simulink model "PMSM_9_yuanlei_SMO_atan_current_step_2019b"  (R2019b)
settings: Solver=ode3  StartTime=0.0  StopTime=0.35  FixedStep=2e-7  RelTol=1e-4  EnableMultiTasking=on
InitFcn:
  | R = 2.8750;
  | L = 8.5e-3;
libraries: powerlib x6, simulink x1
settings Model: Creator=Lei  LastModifiedBy=Administrator
settings DataIOCC: LimitDataPoints=on  SaveFormat=Array  ReturnWorkspaceOutputs=off
settings OptimizationCC: ExpressionDepthLimit=2147483647  InitFltsAndDblsToZero=on  LifeSpan=inf
settings DebuggingCC: SaveWithParameterizedLinksMsg=none  UnderspecifiedInitializationDetection=Classic  MergeDetectMultiDrivingBlocksExec=none  SignalResolutionControl=TryResolveAllWithWarning  SolverPrmCheckMsg=warning  MultiTaskDSMMsg=warning  MultiTaskCondExecSysMsg=none  FcnCallInpInsideContextMsg=warning  UnconnectedLineMsg=none  StateNameClashWarn=warning  SFUnexpectedBacktrackingDiag=warning  SFNoUnconditionalDefaultTransitionDiag=warning  SFExecutionAtInitializationDiag=none  ArithmeticOperatorsInVariantConditions=warning
settings HardwareCC: ProdBitPerPointer=32  ProdBitPerSizeT=32  ProdBitPerPtrDiffT=32  ProdLargestAtomicFloat=None  ProdIntDivRoundTo=Undefined  ProdEndianess=Unspecified  ProdWordSize=32  ProdHWDeviceType=32-bit Generic
settings ModelReferenceCC: PropagateSignalLabelsOutOfModel=off
settings SFSimCC: SimUseLocalCustomCode=off  CustomCodeUndefinedFunction=UseInterfaceOnly
settings RTWCC: RTWUseLocalCustomCode=off
settings CodeAppCC: StateflowObjectComments=on
settings GRTTargetCC: TargetFcnLib=ansi_tfl_tmw.mat  TargetLangStandard=C89/C90 (ANSI)  GeneratePreprocessorConditionals=Disable all  CombineOutputUpdateFcns=off  GRTInterface=on
settings ConfigComp: CovMetricSettings=dw  CovHtmlReporting=on  CovSaveCumulativeToWorkspaceVar=on  CovSaveSingleToWorkspaceVar=on  CovExternalEMLEnable=off  CovSFcnEnable=off
settings SimscapeCC: SimscapeNormalizeSystem=off

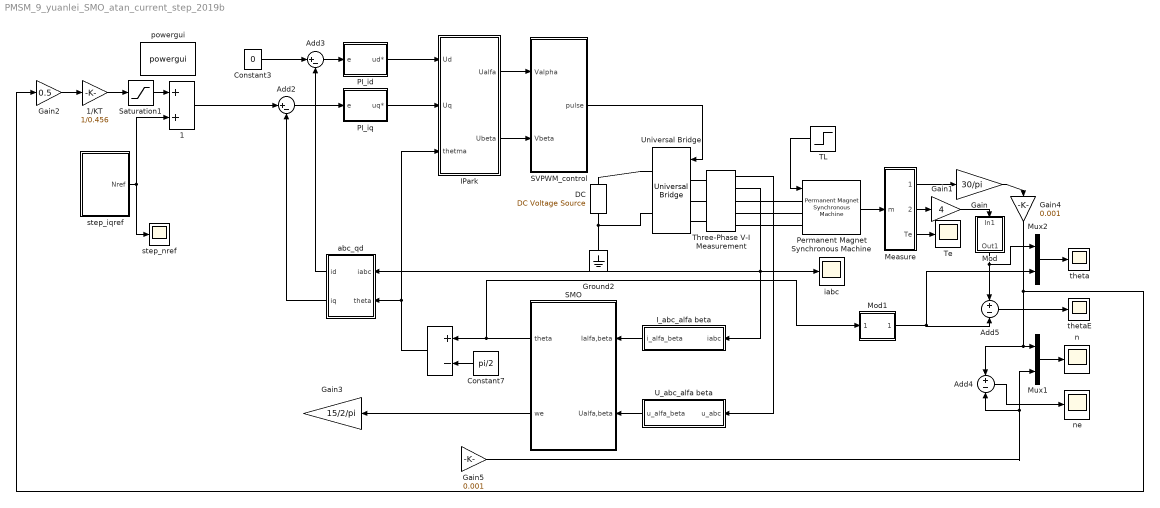
== system PMSM_9_yuanlei_SMO_atan_current_step_2019b ==
  "  " : Sum  Inputs=+-
  "  1" : Sum
  1/KT : Gain  Gain=1/0.456
  Add2 : Sum  Inputs=|+-
  Add3 : Sum  Inputs=|+-
  Add4 : Sum  Inputs=+|-
  Add5 : Sum  Inputs=+|-
  Constant3 : Constant  Value=0
  Constant7 : Constant  Value=pi/2
  "DC " : powerlib/Electrical Sources/DC Voltage Source  Amplitude=311  Measurements=None
      settings: SourceProductName=Simscape Electrical
  Gain : Gain  Gain=30/pi
  Gain1 : Gain  Gain=4
  Gain2 : Gain  Gain=0.5
  Gain3 : Gain  Gain=15/2/pi
  Gain4 : Gain  Gain=0.001
  Gain5 : Gain  Gain=0.001
  Ground2 : powerlib/Elements/Ground  LConnTagsString=a
      settings: SourceProductName=Simscape Electrical
  IPark : Subsystem
  I_abc_alfa beta : Subsystem
  Measure : Subsystem
  Mod : Subsystem
  Mod1 : Subsystem
  Mux1 : Mux  Inputs=2
  Mux2 : Mux  Inputs=2
  PI_id : Subsystem
      mask Display: disp('PI')
  PI_iq : Subsystem
      mask Display: disp('PI')
  Permanent Magnet Synchronous Machine : powerlib/Machines/Permanent Magnet Synchronous Machine  NbPhases=3  FluxDistribution=Sinusoidal  RotorType=Salient-pole  MechanicalLoad=Torque Tm  PresetModel=No  ShowDetailedParameters=on  MeasurementBus=off  Resistance=2.8750  Inductance=8.5e-3  dqInductances=[8.5e-3, 8.5e-3]  La=0.000835  MachineConstant=Flux linkage established by magnets (V.s)  Flux=0.175  VoltageCst=126.966  TorqueCst=1.05  Flat=120  Mechanical="[ 1e-3, 0,  4 ]"  PolePairs=4  InitialConditions=[0,0, 0,0]  InitialConditions5ph=[0 0 0 0 0 0]  RefAngle=90 degrees behind phase A axis (modified Park)  IterativeDiscreteModel=Trapezoidal non iterative  TsBlock=-1  TsPowergui=0
  SMO : Subsystem
  SVPWM_control : Subsystem
  Saturation1 : Saturate  UpperLimit=1  LowerLimit=-1
  TL : Step  Time=0  After=3  SampleTime=0
  Te : Scope
  Three-Phase V-I Measurement : powerlib/Measurements/Three-Phase V-I Measurement  VoltageMeasurement=phase-to-ground  SetLabelV=off  LabelV=Vabc  Vpu=off  VpuLL=off  CurrentMeasurement=yes  SetLabelI=off  LabelI=Iabc  Ipu=off  Pbase=100e6  Vbase=500e3  OutputType=Complex  PhasorSimulation=off  PSBequivalent=0
      settings: SourceProductName=Simscape Electrical
  U_abc_alfa beta : Subsystem
  Universal Bridge : powerlib/Power Electronics/Universal Bridge  Arms=3  SnubberResistance=1e5  SnubberCapacitance=inf  Device=IGBT / Diodes  Ron=1e-3  Lon=0  ForwardVoltages="[  0  0  ]"  ForwardVoltage=0  GTOparameters=[ 10e-6 , 20e-6 ]  IGBTparameters=[ 1e-6 , 2e-6 ]  Measurements=None  Measurements_2=None  converterType=Rectifier
      settings: SourceProductName=Simscape Electrical
  abc_qd : Subsystem
  iabc : Scope
  n : Scope
  ne : Scope
  powergui : powerlib/powergui  Priority=1  SimulationMode=Continuous  SampleTime=50e-6  frequency=60  Iterations=50  frequencyindice=0  Pbase=100e6  ErrMax=1e-4  UnitsV=kV  UnitsW=MW  buscounter=0  FunctionMessages=off  echomessages=off  EnableUseOfTLC=off  CurrentSourceSwitches=off  DisableSnubberDevices=off  DisableRonSwitches=off  DisableVfSwitches=off  DisplayEquations=off  AutomaticDiscreteSolvers=off  SolverType=Tustin/Backward Euler (TBE)  Interpol=off  ExternalGateDelay=off  methode=off  Ts=100  x0status=blocks  SPID=off  SwTol=0  HookPort=off  NonlinearTolerance=1e-4  nMaxIteration=100  ContinueOnMaxIteration=off  RestoreLinks=warning  ResistiveCurrentMeasurement=off  Frange=[0:2:500]  Ylog=off  Xlog=on  ShowGrid=off  save=off  variable=ZData  structure=0  ZoomFFT=off  StartTime=0.0  cycles=1  DisplayStyle=1  fundamental=60  FreqAxis=off  MaxFrequency=1000  frequencyindicesteady=1  RmsSteady=1  display=off
      settings: SourceProductName=Simscape Electrical
  step_iqref : Subsystem
  step_nref : Scope
  theta : Scope
  thetaE : Scope
  wires:
  Constant3/1 -> Add3/1
  SVPWM_control/1(pulse) -> Universal Bridge/1
  IPark/1(Ualfa) -> SVPWM_control/1(Valpha)
  IPark/2(Ubeta) -> SVPWM_control/2(Vbeta)
  PI_iq/1(uq*) -> IPark/2(Uq)
  TL/1 -> Permanent Magnet Synchronous Machine/1
  "  1"/1 -> Add2/1
  SMO/2(we) -> Gain3/1
  Permanent Magnet Synchronous Machine/1 -> Measure/1(m)
  Measure/1(wm) -> Gain/1
  Measure/2(The) -> Gain1/1
  Measure/3(Te) -> Te/1
  Three-Phase V-I Measurement/1 -> U_abc_alfa beta/1(u_abc)
  Add2/1 -> PI_iq/1(e)
  Add3/1 -> PI_id/1(e)
  PI_id/1(ud*) -> IPark/1(Ud)
  abc_qd/1(id) -> Add3/2
  abc_qd/2(iq) -> Add2/2
  I_abc_alfa beta/1(i_alfa_beta) -> SMO/1(Ialfa,beta)
  U_abc_alfa beta/1(u_alfa_beta) -> SMO/2(Ualfa,beta)
  Constant7/1 -> "  "/2
  "  "/1 -> IPark/3(thetma), abc_qd/2(theta)
  Three-Phase V-I Measurement/2 -> abc_qd/1(iabc), iabc/1, I_abc_alfa beta/1(iabc)
  Mux1/1 -> n/1
  Gain/1 -> Gain4/1
  Gain1/1 -> Mod/1(In1)
  Mux2/1 -> theta/1
  SMO/1(theta) -> Mod1/1(In1), "  "/1
  Add5/1 -> thetaE/1
  Add4/1 -> ne/1
  Mod/1(Out1) -> Mux2/1, Add5/1
  Mod1/1(Out1) -> Add5/2, Mux2/2
  step_iqref/1(Nref) -> "  1"/2, step_nref/1
  Gain2/1 -> 1/KT/1
  Gain4/1 -> Add4/1, Mux1/1, Gain2/1
  Gain5/1 -> Add4/2, Mux1/2
  1/KT/1 -> Saturation1/1
  Saturation1/1 -> "  1"/1
  connections:
  Universal Bridge/RConn1 -- "DC "/RConn1
  "DC "/LConn1 -- Ground2/LConn1 -- Universal Bridge/RConn2
  Universal Bridge/LConn1 -- Three-Phase V-I Measurement/LConn1
  Universal Bridge/LConn2 -- Three-Phase V-I Measurement/LConn2
  Universal Bridge/LConn3 -- Three-Phase V-I Measurement/LConn3
  Three-Phase V-I Measurement/RConn1 -- Permanent Magnet Synchronous Machine/LConn1
  Three-Phase V-I Measurement/RConn2 -- Permanent Magnet Synchronous Machine/LConn2
  Three-Phase V-I Measurement/RConn3 -- Permanent Magnet Synchronous Machine/LConn3

== system PMSM_9_yuanlei_SMO_atan_current_step_2019b/IPark ==
  Ud : Inport
  Uq : Inport  Port=2
  thetma : Inport  Port=3
  Fcn : Fcn  Expr=cos(u[3])*u[2]-sin(u[3])*u[1]
  Fcn1 : Fcn  Expr=sin(u[3])*u[2]+cos(u[3])*u[1]
  Mux : Mux  Inputs=3
  Ualfa : Outport
  Ubeta : Outport  Port=2
  wires:
  Uq/1 -> Mux/1
  Ud/1 -> Mux/2
  thetma/1 -> Mux/3
  Mux/1 -> Fcn/1, Fcn1/1
  Fcn/1 -> Ualfa/1
  Fcn1/1 -> Ubeta/1

== system PMSM_9_yuanlei_SMO_atan_current_step_2019b/I_abc_alfa beta ==
  iabc : Inport
  Fcn : Fcn  Expr=(2*u(1)-u(2)-u(3))/3
  Fcn1 : Fcn  Expr=(u(2)-u(3))/(3^(1/2))
  Mux2 : Mux  Inputs=2
  i_alfa_beta : Outport
  wires:
  iabc/1 -> Fcn/1, Fcn1/1
  Mux2/1 -> i_alfa_beta/1
  Fcn/1 -> Mux2/1
  Fcn1/1 -> Mux2/2

== system PMSM_9_yuanlei_SMO_atan_current_step_2019b/Measure ==
  m : Inport
  Bus Selector1 : BusSelector  OutputSignals=Rotor speed wm (rad/s),Rotor angle thetam (rad),Electromagnetic torque Te (N*m)
  wm : Outport
  The : Outport  Port=2
  Te : Outport  Port=3
  wires:
  Bus Selector1/2 -> The/1  "<Rotor angle thetam (rad)>"
  Bus Selector1/3 -> Te/1  "<Electromagnetic torque Te (N*m)>"
  m/1 -> Bus Selector1/1
  Bus Selector1/1 -> wm/1  "<Rotor speed wm (rad/s)>"

== system PMSM_9_yuanlei_SMO_atan_current_step_2019b/Mod ==
  In1 : Inport
  Constant1 : Constant  Value=pi/4
  Math Function : Math  Operator=mod  SaturateOnIntegerOverflow=on
  Out1 : Outport
  wires:
  Constant1/1 -> Math Function/2
  Math Function/1 -> Out1/1
  In1/1 -> Math Function/1

== system PMSM_9_yuanlei_SMO_atan_current_step_2019b/Mod1 ==
  In1 : Inport
  Constant1 : Constant  Value=pi/4
  Math Function : Math  Operator=mod  SaturateOnIntegerOverflow=on
  Out1 : Outport
  wires:
  In1/1 -> Math Function/1
  Math Function/1 -> Out1/1
  Constant1/1 -> Math Function/2

== system PMSM_9_yuanlei_SMO_atan_current_step_2019b/PI_id ==
  e : Inport
  Add : Sum
  Integrator : Integrator
  Ki : Gain  Gain=R*2000
  Kp : Gain  Gain=L*2000
  Saturation : Saturate  UpperLimit=350  LowerLimit=-350
  ud* : Outport
  wires:
  Ki/1 -> Integrator/1
  e/1 -> Kp/1, Ki/1
  Saturation/1 -> ud*/1
  Integrator/1 -> Add/2
  Kp/1 -> Add/1
  Add/1 -> Saturation/1

== system PMSM_9_yuanlei_SMO_atan_current_step_2019b/PI_iq ==
  e : Inport
  Add : Sum
  Integrator : Integrator
  Ki : Gain  Gain=R*2000
  Kp : Gain  Gain=L*2000
  Saturation : Saturate  UpperLimit=350  LowerLimit=-350
  uq* : Outport
  wires:
  Ki/1 -> Integrator/1
  e/1 -> Kp/1, Ki/1
  Saturation/1 -> uq*/1
  Integrator/1 -> Add/2
  Kp/1 -> Add/1
  Add/1 -> Saturation/1

== system PMSM_9_yuanlei_SMO_atan_current_step_2019b/SMO ==
  Ialfa,beta : Inport
  Ualfa,beta : Inport  Port=2
  Arctan_function : Subsystem
  SMO : Subsystem
  theta : Outport
  we : Outport  Port=2
  wires:
  Ualfa,beta/1 -> SMO/1(Ualfa,beta)
  Ialfa,beta/1 -> SMO/2(Ialfa,beta)
  SMO/1(Ealpha^) -> Arctan_function/1(Ealpha^)
  SMO/2(Ebeta^) -> Arctan_function/2(Ebeta^)
  Arctan_function/1(theta) -> theta/1
  Arctan_function/2(we) -> we/1

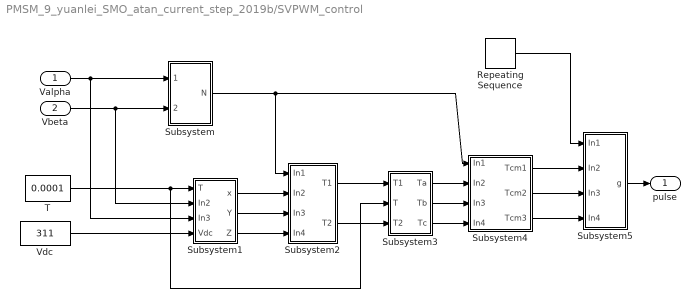
== system PMSM_9_yuanlei_SMO_atan_current_step_2019b/SVPWM_control ==
  Valpha : Inport
  Vbeta : Inport  Port=2
  Repeating Sequence : simulink/Sources/Repeating Sequence  rep_seq_t=[0 0.0001 0.0002]  rep_seq_y=[0 0.0001 0]
  Subsystem : Subsystem
  Subsystem1 : Subsystem
  Subsystem2 : Subsystem
  Subsystem3 : Subsystem
  Subsystem4 : Subsystem
  Subsystem5 : Subsystem
  T : Constant  Value=0.0001
  Vdc : Constant  Value=311
  pulse : Outport
  wires:
  Subsystem5/1(g) -> pulse/1
  Repeating Sequence/1 -> Subsystem5/1(In1)
  Subsystem4/3(Tcm3) -> Subsystem5/4(In4)
  Subsystem4/2(Tcm2) -> Subsystem5/3(In3)
  Subsystem4/1(Tcm1) -> Subsystem5/2(In2)
  Subsystem3/3(Tc) -> Subsystem4/4(In4)
  Subsystem3/2(Tb) -> Subsystem4/3(In3)
  Subsystem3/1(Ta) -> Subsystem4/2(In2)
  Subsystem2/2(T2) -> Subsystem3/3(T2)
  Subsystem2/1(T1) -> Subsystem3/1(T1)
  Subsystem1/3(Z) -> Subsystem2/4(In4)
  Subsystem1/2(Y) -> Subsystem2/3(In3)
  Subsystem1/1(x) -> Subsystem2/2(In2)
  Subsystem/1(N) -> Subsystem4/1(In1), Subsystem2/1(In1)
  Vdc/1 -> Subsystem1/4(Vdc)
  T/1 -> Subsystem3/2(T), Subsystem1/1(T)
  Vbeta/1 -> Subsystem1/2(In2), Subsystem/2(Vbeta)
  Valpha/1 -> Subsystem1/3(In3), Subsystem/1(Valpha)

== system PMSM_9_yuanlei_SMO_atan_current_step_2019b/U_abc_alfa beta ==
  u_abc : Inport
  Fcn : Fcn  Expr=(2*u(1)-u(2)-u(3))/3
  Fcn1 : Fcn  Expr=(u(2)-u(3))/(3^(1/2))
  Mux2 : Mux  Inputs=2
  u_alfa_beta : Outport
  wires:
  u_abc/1 -> Fcn/1, Fcn1/1
  Mux2/1 -> u_alfa_beta/1
  Fcn/1 -> Mux2/1
  Fcn1/1 -> Mux2/2

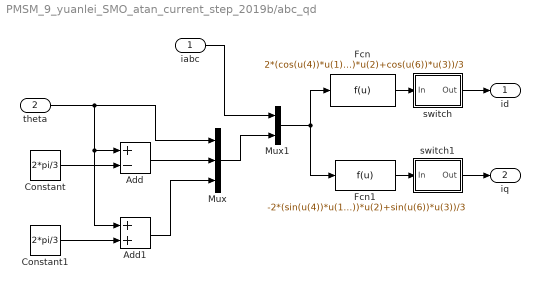
== system PMSM_9_yuanlei_SMO_atan_current_step_2019b/abc_qd ==
  iabc : Inport
  theta : Inport  Port=2
  Add : Sum  Inputs=+-
  Add1 : Sum
  Constant : Constant  Value=2*pi/3
  Constant1 : Constant  Value=2*pi/3
  Fcn : Fcn  Expr=2*(cos(u(4))*u(1)+cos(u(5))*u(2)+cos(u(6))*u(3))/3
  Fcn1 : Fcn  Expr=-2*(sin(u(4))*u(1)+sin(u(5))*u(2)+sin(u(6))*u(3))/3
  Mux : Mux  Inputs=3
  Mux1 : Mux  Inputs=2
  switch : Subsystem
  switch1 : Subsystem
  id : Outport
  iq : Outport  Port=2
  wires:
  Constant1/1 -> Add1/2
  Constant/1 -> Add/2
  theta/1 -> Mux/1, Add1/1, Add/1
  Add/1 -> Mux/2
  Add1/1 -> Mux/3
  Mux/1 -> Mux1/2
  iabc/1 -> Mux1/1
  Mux1/1 -> Fcn/1, Fcn1/1
  Fcn/1 -> switch/1(In)
  switch/1(Out) -> id/1
  Fcn1/1 -> switch1/1(In)
  switch1/1(Out) -> iq/1

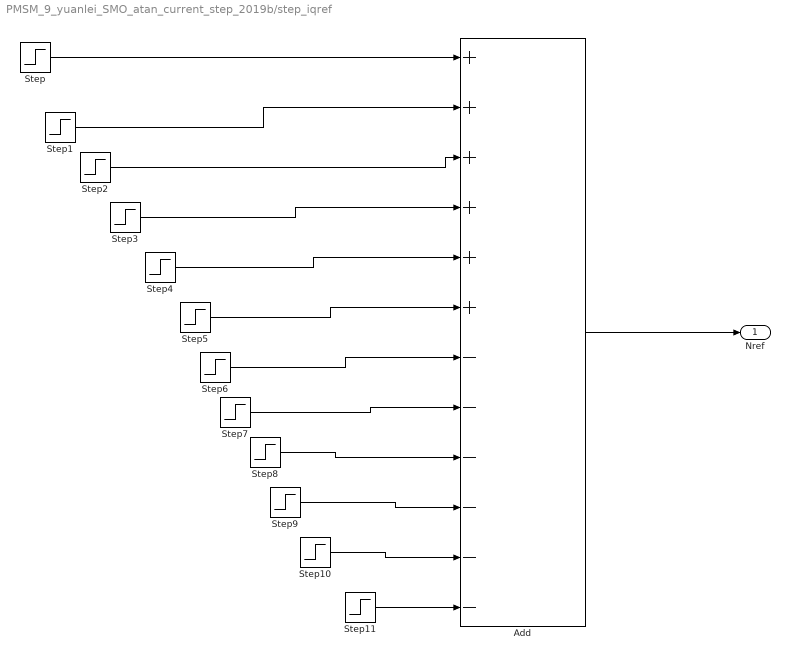
== system PMSM_9_yuanlei_SMO_atan_current_step_2019b/step_iqref ==
  Add : Sum  Inputs=++++++------
  Step : Step  Time=0.025  Before=0.00001  After=0.5  SampleTime=0
  Step1 : Step  Time=0.05  After=0.5  SampleTime=0
  Step10 : Step  Time=0.275  After=0.5  SampleTime=0
  Step11 : Step  Time=0.3  After=0.499999  SampleTime=0
  Step2 : Step  Time=0.075  After=0.5  SampleTime=0
  Step3 : Step  Time=0.1  After=0.5  SampleTime=0
  Step4 : Step  Time=0.125  After=0.5  SampleTime=0
  Step5 : Step  Time=0.15  After=0.5  SampleTime=0
  Step6 : Step  Time=0.175  After=0.5  SampleTime=0
  Step7 : Step  Time=0.2  After=0.5  SampleTime=0
  Step8 : Step  Time=0.225  After=0.5  SampleTime=0
  Step9 : Step  Time=0.25  After=0.5  SampleTime=0
  Nref : Outport
  wires:
  Step/1 -> Add/1
  Step1/1 -> Add/2
  Step2/1 -> Add/3
  Step3/1 -> Add/4
  Step4/1 -> Add/5
  Step5/1 -> Add/6
  Step6/1 -> Add/7
  Step7/1 -> Add/8
  Step8/1 -> Add/9
  Step9/1 -> Add/10
  Step10/1 -> Add/11
  Step11/1 -> Add/12
  Add/1 -> Nref/1

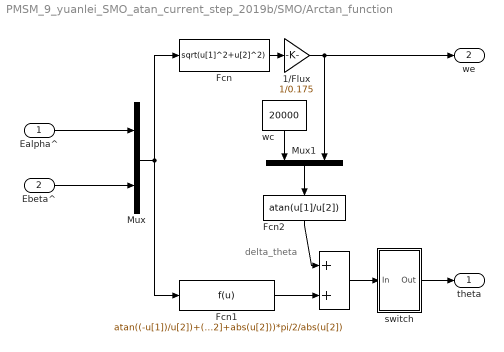
== system PMSM_9_yuanlei_SMO_atan_current_step_2019b/SMO/Arctan_function ==
  note: delta_theta
  Ealpha^ : Inport
  Ebeta^ : Inport  Port=2
  "  " : Sum
  1/Flux : Gain  Gain=1/0.175
  Fcn : Fcn  Expr=sqrt(u[1]^2+u[2]^2)
  Fcn1 : Fcn  Expr=atan((-u[1])/u[2])+(-u[2]+abs(u[2]))*pi/2/abs(u[2])
  Fcn2 : Fcn  Expr=atan(u[1]/u[2])
  Mux : Mux  Inputs=2
  Mux1 : Mux  Inputs=2
  switch : Subsystem
  wc : Constant  Value=20000
  theta : Outport
  we : Outport  Port=2
  wires:
  Mux/1 -> Fcn/1, Fcn1/1
  Fcn/1 -> 1/Flux/1
  1/Flux/1 -> we/1, Mux1/2
  Fcn1/1 -> "  "/2
  "  "/1 -> switch/1(In)
  Mux1/1 -> Fcn2/1
  Fcn2/1 -> "  "/1
  wc/1 -> Mux1/1
  switch/1(Out) -> theta/1
  Ebeta^/1 -> Mux/2
  Ealpha^/1 -> Mux/1

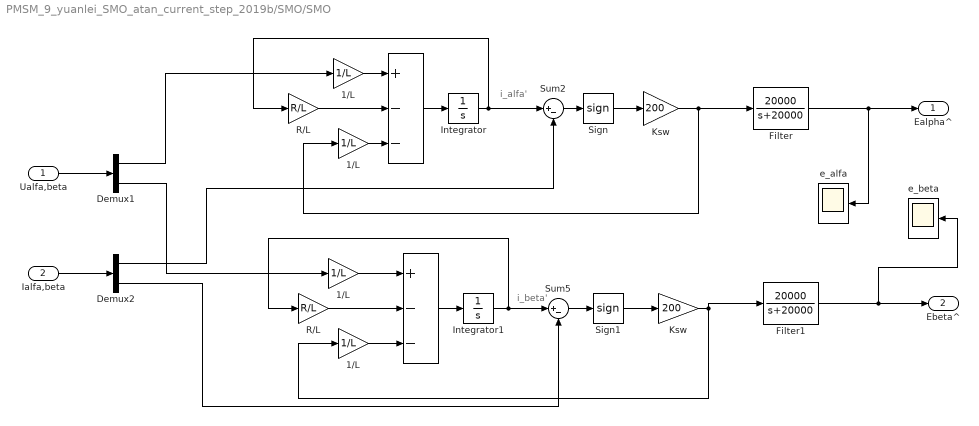
== system PMSM_9_yuanlei_SMO_atan_current_step_2019b/SMO/SMO ==
  note: i_alfa'
  note: i_beta'
  Ualfa,beta : Inport
  Ialfa,beta : Inport  Port=2
  " " : Sum  Inputs=+--
  "   " : Sum  Inputs=+--
  " 1/L" : Gain  Gain=1/L
  " 1/L " : Gain  Gain=1/L
  1/L : Gain  Gain=1/L
  "1/L " : Gain  Gain=1/L
  Demux1 : Demux  Outputs=2
  Demux2 : Demux  Outputs=2
  Filter : TransferFcn  Numerator=[20000]  Denominator=[1 20000]
  Filter1 : TransferFcn  Numerator=[20000]  Denominator=[1 20000]
  Integrator : Integrator
  Integrator1 : Integrator
  Ksw : Gain  Gain=200
  "Ksw " : Gain  Gain=200
  R/L : Gain  Gain=R/L
  "R/L " : Gain  Gain=R/L
  Sign : Signum  ZeroCross=off
  Sign1 : Signum  ZeroCross=off
  Sum2 : Sum  Inputs=|+-
  Sum5 : Sum  Inputs=|+-
  e_alfa : Scope
  e_beta : Scope
  Ealpha^ : Outport
  Ebeta^ : Outport  Port=2
  wires:
  Integrator/1 -> Sum2/1, R/L/1
  Sign/1 -> Ksw/1
  Ksw/1 -> "1/L "/1, Filter/1
  Integrator1/1 -> Sum5/1, "R/L "/1
  Sum5/1 -> Sign1/1
  Sign1/1 -> "Ksw "/1
  "Ksw "/1 -> " 1/L "/1, Filter1/1
  Demux2/1 -> Sum2/2
  Demux2/2 -> Sum5/2
  1/L/1 -> " "/1
  R/L/1 -> " "/2
  "1/L "/1 -> " "/3
  " "/1 -> Integrator/1
  Demux1/2 -> " 1/L"/1
  " 1/L"/1 -> "   "/1
  "R/L "/1 -> "   "/2
  "   "/1 -> Integrator1/1
  " 1/L "/1 -> "   "/3
  Sum2/1 -> Sign/1
  Filter1/1 -> e_beta/1, Ebeta^/1
  Filter/1 -> Ealpha^/1, e_alfa/1
  Demux1/1 -> 1/L/1
  Ialfa,beta/1 -> Demux2/1
  Ualfa,beta/1 -> Demux1/1

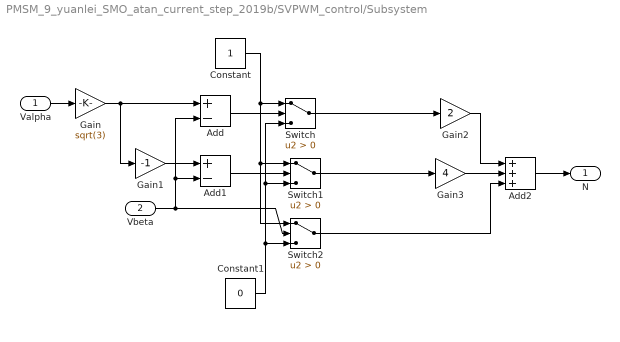
== system PMSM_9_yuanlei_SMO_atan_current_step_2019b/SVPWM_control/Subsystem ==
  Valpha : Inport
  Vbeta : Inport  Port=2
  Add : Sum  Inputs=+-
  Add1 : Sum  Inputs=+-
  Add2 : Sum  Inputs=+++
  Constant : Constant
  Constant1 : Constant  Value=0
  Gain : Gain  Gain=sqrt(3)
  Gain1 : Gain  Gain=-1
  Gain2 : Gain  Gain=2
  Gain3 : Gain  Gain=4
  Switch : Switch  Criteria=u2 > Threshold
  Switch1 : Switch  Criteria=u2 > Threshold
  Switch2 : Switch  Criteria=u2 > Threshold
  N : Outport
  wires:
  Valpha/1 -> Gain/1
  Gain3/1 -> Add2/2
  Gain2/1 -> Add2/1
  Add1/1 -> Switch1/2
  Gain1/1 -> Add1/1
  Switch1/1 -> Gain3/1
  Switch2/1 -> Add2/3
  Switch/1 -> Gain2/1
  Add/1 -> Switch/2
  Gain/1 -> Gain1/1, Add/1
  Constant1/1 -> Switch/3, Switch1/3, Switch2/3
  Constant/1 -> Switch1/1, Switch2/1, Switch/1
  Vbeta/1 -> Add1/2, Add/2, Switch2/2
  Add2/1 -> N/1

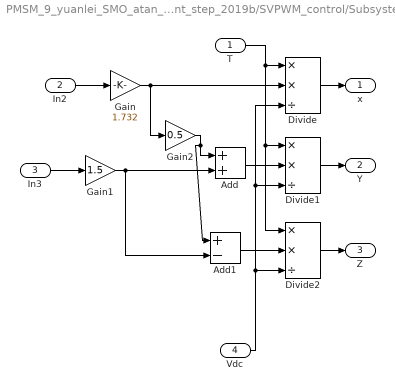
== system PMSM_9_yuanlei_SMO_atan_current_step_2019b/SVPWM_control/Subsystem1 ==
  T : Inport
  In2 : Inport  Port=2
  In3 : Inport  Port=3
  Vdc : Inport  Port=4
  Add : Sum
  Add1 : Sum  Inputs=+-
  Divide : Product  Inputs=**/
  Divide1 : Product  Inputs=**/
  Divide2 : Product  Inputs=**/
  Gain : Gain  Gain=1.732
  Gain1 : Gain  Gain=1.5
  Gain2 : Gain  Gain=0.5
  x : Outport
  Y : Outport  Port=2
  Z : Outport  Port=3
  wires:
  Divide2/1 -> Z/1
  Divide1/1 -> Y/1
  Divide/1 -> x/1
  In3/1 -> Gain1/1
  In2/1 -> Gain/1
  Add1/1 -> Divide2/2
  Add/1 -> Divide1/2
  Gain1/1 -> Add1/2, Add/2
  Gain2/1 -> Add1/1, Add/1
  Gain/1 -> Gain2/1, Divide/2
  Vdc/1 -> Divide/3, Divide1/3, Divide2/3
  T/1 -> Divide2/1, Divide1/1, Divide/1

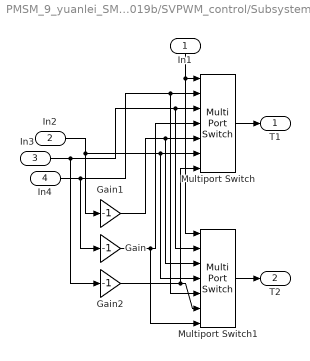
== system PMSM_9_yuanlei_SMO_atan_current_step_2019b/SVPWM_control/Subsystem2 ==
  In1 : Inport
  In2 : Inport  Port=2
  In3 : Inport  Port=3
  In4 : Inport  Port=4
  Gain : Gain  Gain=-1
  Gain1 : Gain  Gain=-1
  Gain2 : Gain  Gain=-1
  Multiport Switch : MultiPortSwitch  Inputs=6
  Multiport Switch1 : MultiPortSwitch  Inputs=6
  T1 : Outport
  T2 : Outport  Port=2
  wires:
  Multiport Switch1/1 -> T2/1
  Multiport Switch/1 -> T1/1
  Gain2/1 -> Multiport Switch/7, Multiport Switch1/6
  Gain1/1 -> Multiport Switch1/3, Multiport Switch/5
  In2/1 -> Gain1/1, Multiport Switch/6, Multiport Switch1/4
  Gain/1 -> Multiport Switch1/7, Multiport Switch/4
  In3/1 -> Gain2/1, Multiport Switch1/2, Multiport Switch/3
  In4/1 -> Gain/1, Multiport Switch/2, Multiport Switch1/5
  In1/1 -> Multiport Switch/1, Multiport Switch1/1

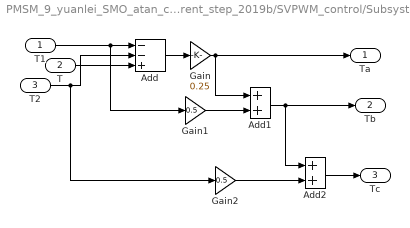
== system PMSM_9_yuanlei_SMO_atan_current_step_2019b/SVPWM_control/Subsystem3 ==
  T1 : Inport
  T : Inport  Port=2
  T2 : Inport  Port=3
  Add : Sum  Inputs=--+
  Add1 : Sum
  Add2 : Sum
  Gain : Gain  Gain=0.25
  Gain1 : Gain  Gain=0.5
  Gain2 : Gain  Gain=0.5
  Ta : Outport
  Tb : Outport  Port=2
  Tc : Outport  Port=3
  wires:
  T/1 -> Add/3
  Add2/1 -> Tc/1
  Gain2/1 -> Add2/2
  Add1/1 -> Add2/1, Tb/1
  Gain1/1 -> Add1/2
  Gain/1 -> Add1/1, Ta/1
  Add/1 -> Gain/1
  T2/1 -> Add/2, Gain2/1
  T1/1 -> Add/1, Gain1/1

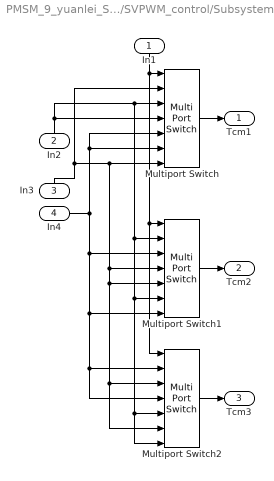
== system PMSM_9_yuanlei_SMO_atan_current_step_2019b/SVPWM_control/Subsystem4 ==
  In1 : Inport
  In2 : Inport  Port=2
  In3 : Inport  Port=3
  In4 : Inport  Port=4
  Multiport Switch : MultiPortSwitch  Inputs=6
  Multiport Switch1 : MultiPortSwitch  Inputs=6
  Multiport Switch2 : MultiPortSwitch  Inputs=6
  Tcm1 : Outport
  Tcm2 : Outport  Port=2
  Tcm3 : Outport  Port=3
  wires:
  Multiport Switch2/1 -> Tcm3/1
  Multiport Switch1/1 -> Tcm2/1
  Multiport Switch/1 -> Tcm1/1
  In1/1 -> Multiport Switch2/1, Multiport Switch1/1, Multiport Switch/1
  In4/1 -> Multiport Switch1/3, Multiport Switch1/7, Multiport Switch2/2, Multiport Switch2/4, Multiport Switch/5, Multiport Switch/6
  In2/1 -> Multiport Switch/4, Multiport Switch/3, Multiport Switch1/2, Multiport Switch1/6, Multiport Switch2/5, Multiport Switch2/7
  In3/1 -> Multiport Switch/2, Multiport Switch/7, Multiport Switch1/4, Multiport Switch1/5, Multiport Switch2/3, Multiport Switch2/6

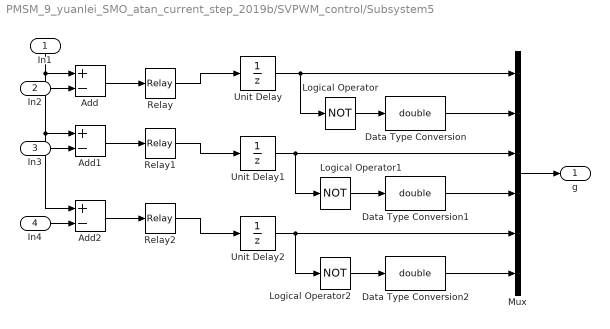
== system PMSM_9_yuanlei_SMO_atan_current_step_2019b/SVPWM_control/Subsystem5 ==
  In1 : Inport
  In2 : Inport  Port=2
  In3 : Inport  Port=3
  In4 : Inport  Port=4
  Add : Sum  Inputs=+-
  Add1 : Sum  Inputs=+-
  Add2 : Sum  Inputs=+-
  Data Type Conversion : DataTypeConversion  OutDataTypeStr=double
  Data Type Conversion1 : DataTypeConversion  OutDataTypeStr=double
  Data Type Conversion2 : DataTypeConversion  OutDataTypeStr=double
  Logical Operator : Logic  Operator=NOT  AllPortsSameDT=off  OutDataTypeStr=boolean
  Logical Operator1 : Logic  Operator=NOT  AllPortsSameDT=off  OutDataTypeStr=boolean
  Logical Operator2 : Logic  Operator=NOT  AllPortsSameDT=off  OutDataTypeStr=boolean
  Mux : Mux  Inputs=6
  Relay : Relay  OffSwitchValue=-eps
  Relay1 : Relay  OffSwitchValue=-eps
  Relay2 : Relay  OffSwitchValue=-eps
  Unit Delay : UnitDelay  SampleTime=-1  HasFrameUpgradeWarning=on
  Unit Delay1 : UnitDelay  SampleTime=-1  HasFrameUpgradeWarning=on
  Unit Delay2 : UnitDelay  SampleTime=-1  HasFrameUpgradeWarning=on
  g : Outport
  wires:
  In4/1 -> Add2/2
  In3/1 -> Add1/2
  In2/1 -> Add/2
  Relay2/1 -> Unit Delay2/1
  Relay1/1 -> Unit Delay1/1
  Relay/1 -> Unit Delay/1
  Unit Delay2/1 -> Mux/5, Logical Operator2/1
  Unit Delay1/1 -> Mux/3, Logical Operator1/1
  Unit Delay/1 -> Logical Operator/1, Mux/1
  Mux/1 -> g/1
  Data Type Conversion/1 -> Mux/2
  Data Type Conversion1/1 -> Mux/4
  Data Type Conversion2/1 -> Mux/6
  Logical Operator2/1 -> Data Type Conversion2/1
  Logical Operator1/1 -> Data Type Conversion1/1
  Logical Operator/1 -> Data Type Conversion/1
  Add1/1 -> Relay1/1
  Add2/1 -> Relay2/1
  Add/1 -> Relay/1
  In1/1 -> Add/1, Add2/1, Add1/1

== system PMSM_9_yuanlei_SMO_atan_current_step_2019b/abc_qd/switch ==
  In : Inport
  Constant4 : Constant  Value=0
  Step1 : Step  Time=0.001  SampleTime=0
  Switch : Switch  Threshold=1
  Out : Outport
  wires:
  Step1/1 -> Switch/2
  Constant4/1 -> Switch/3
  In/1 -> Switch/1
  Switch/1 -> Out/1

== system PMSM_9_yuanlei_SMO_atan_current_step_2019b/abc_qd/switch1 ==
  In : Inport
  Constant4 : Constant  Value=0
  Step1 : Step  Time=0.001  SampleTime=0
  Switch : Switch  Threshold=1
  Out : Outport
  wires:
  Switch/1 -> Out/1
  In/1 -> Switch/1
  Constant4/1 -> Switch/3
  Step1/1 -> Switch/2

== system PMSM_9_yuanlei_SMO_atan_current_step_2019b/SMO/Arctan_function/switch ==
  In : Inport
  Constant4 : Constant  Value=0
  Step1 : Step  Time=0.001  SampleTime=0
  Switch : Switch  Threshold=1
  Out : Outport
  wires:
  Step1/1 -> Switch/2
  Constant4/1 -> Switch/3
  In/1 -> Switch/1
  Switch/1 -> Out/1
